simulink model "uniqueWordMethod"  (R2018b)
settings: Solver=FixedStepDiscrete  StartTime=0.0  StopTime=1000  RelTol=1e-3
libraries: simulink x2, commutil2 x2, commdigbbndpm3 x2, commfilt2 x2, dspstat3 x1, commrandsrc3 x1, commsink2 x1, commrflib2 x1, dspsigops x1
settings Model: Creator=sikor  LastModifiedBy=sikor
settings OptimizationCC: LifeSpan=inf
settings DebuggingCC: SFUnexpectedBacktrackingDiag=warning  SFNoUnconditionalDefaultTransitionDiag=warning
settings SFSimCC: SimUseLocalCustomCode=off
settings RTWCC: RTWUseLocalCustomCode=off
settings CodeAppCC: StateflowObjectComments=on
settings GRTTargetCC: TargetLangStandard=C89/C90 (ANSI)  GeneratePreprocessorConditionals=Disable all
settings ConfigComp: CovMetricSettings=dw  CovHtmlReporting=on  CovSaveCumulativeToWorkspaceVar=on  CovSaveSingleToWorkspaceVar=on  CovExternalEMLEnable=off

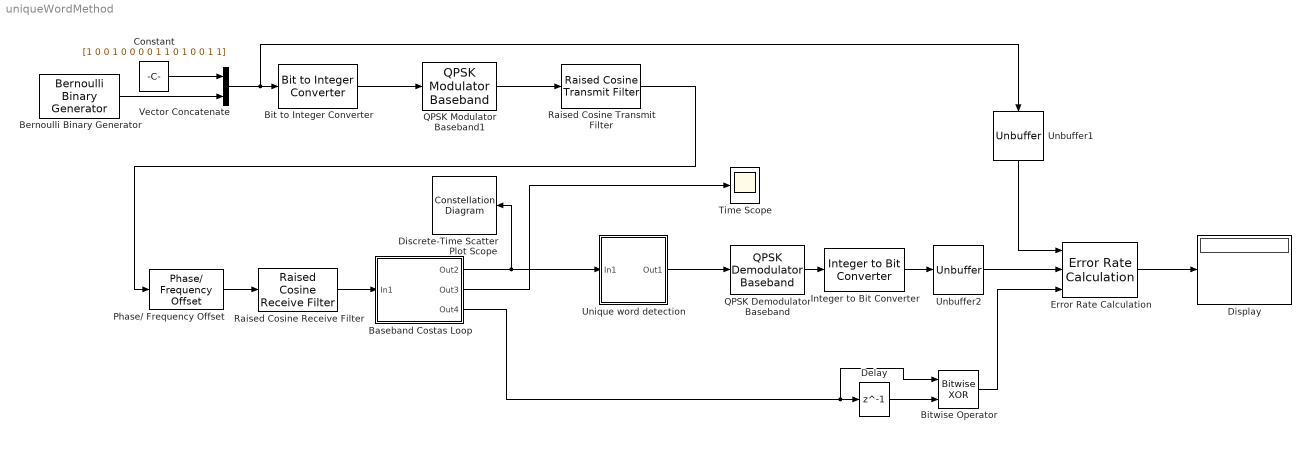
== system uniqueWordMethod ==
  Baseband Costas Loop : Subsystem  mask{loopBw=2.0*pi/100.0, sampleTime=1}
      mask prompts: loopBw "Select loop bandwidth"; sampleTime "Sample time"
      mask init:
      | damp=0.707;
      | %set_param('costasLoop','AlgebraicLoopSolver','TrustRegion')
      | alpha = (4.0 * damp * loopBw) / (1.0 + 2.0 * damp * loopBw + loopBw * loopBw); 
      | beta = (4.0 * loopBw * loopBw) / (1.0 + 2.0 * damp * loopBw + loopBw * loopBw); 
      | set_param(sprintf('%s/Baseband Costas Loop/Alfa',gcs),'Gain',sprintf('%f',alpha))
      | set_param(sprintf('%s/Baseband Costas Loop/Beta',gcs),'Gain',sprintf('%f',beta))
      | %set_param(sprintf('%s/Baseband Costas Loop/Mean1',gcs),'Ts',sprintf('%f',sampleTime))
      mask Display: disp('Costas\nLoop');
  Bernoulli Binary Generator : commrandsrc3/Bernoulli Binary Generator  ProbabilityOfZero=0.5  SeedSource=Auto  Seed=0  SampleTime=128  SamplesPerFrame=240  OutputDataType=uint8  SimulateUsing=Interpreted execution
      settings: SourceProductName=Communications Toolbox
  Bit to Integer Converter : commutil2/Bit to Integer Converter  nbits=2  bitOrder=MSB first  signedOutputValues=Unsigned  outDtype=int16  outDtypeSigned=Inherit via internal rule
      settings: SourceProductName=Communications Toolbox
  Bitwise Operator : simulink/Logic and Bit Operations/Bitwise Operator  logicop=XOR  UseBitMask=off  NumInputPorts=2  BitMask=bin2dec('11011001')  BitMaskRealWorld=Stored Integer
  Constant : Constant  Value=[1 0 0 1 0 0 0 0 1 1 0 1 0 0 1 1]  OutDataTypeStr=uint8  SampleTime=128
  Delay : Delay  DelayLength=1  InitialCondition=0
  Discrete-Time Scatter Plot Scope : ConstellationDiagram  Tag=ScatterPlot
  Display : Display
  Error Rate Calculation : commsink2/Error Rate Calculation  N=276  st_delay=0  cp_mode=Entire frame  subframe=[]  PMode=Port  WsName=ErrorVec  RsMode2=on  stop=off  numErr=100  maxBits=1e6
      settings: SourceProductName=Communications Toolbox
  Integer to Bit Converter : commutil2/Integer to Bit Converter  nbits=2  signedInputValues=Unsigned  bitOrder=MSB first  outDtype=Inherit via internal rule
      settings: SourceProductName=Communications Toolbox
  Phase/ Frequency Offset : commrflib2/Phase// Frequency Offset  phaseOffset=40  freqPort=off  freqOffset=.0000000000000000045
      settings: SourceProductName=Communications Toolbox
  QPSK Demodulator Baseband : commdigbbndpm3/QPSK Demodulator Baseband  OutType=Integer  DecType=Hard decision  VarSource=Dialog  Variance=1  Dec=Gray  Ph=pi/4  outDtype1=Inherit via internal rule  outDtype2=int16  derotateFactorWordLen=16  derotateFactorDataTypeStr=Inherit: Same word length as input  derotateFactorLastDataTypeStr=Inherit: Same word length as input
      settings: SourceProductName=Communications Toolbox
  QPSK Modulator Baseband1 : commdigbbndpm3/QPSK Modulator Baseband  InType=Integer  Enc=Gray  Ph=pi/4  outDtype=double  outWordLen=16  outUDDataType=sfix(16)  outFracLenMode=Best precision  outFracLen=15  outDataTypeStr=double  outLastDataTypeStr=double
      settings: SourceProductName=Communications Toolbox
  Raised Cosine Receive Filter : commfilt2/Raised Cosine Receive Filter  filtType=Square root  R=0.2  filtSpan=10  N=4  downFactor=4  downOffset=0  filterGain=1  InputProcessing=Columns as channels (frame based)  RateOptions=Allow multirate processing  framing=Mute  checkCoeff=off  variableName=rcRxFilt  currentFiltSpan=10  D=5  inputOffset=0  sampMode=Mute  saveAsFlag=0  rateMode=Downsampling  checkGain=Normalized  launchFVT=on  roundingMode=Floor  overflowMode=off  coeffDataTypeStr=Inherit: Same word length as input  coeffMin=[]  coeffMax=[]  coeffLastDataTypeStr=Inherit: Same word length as input  accumDataTypeStr=Inherit: Same as product output  accumLastDataTypeStr=Inherit: Same as product output  outputDataTypeStr=Inherit: Same as accumulator  outputMin=[]  outputMax=[]  outputLastDataTypeStr=Inherit: Same as accumulator
      settings: SourceProductName=Communications Toolbox
  Raised Cosine Transmit Filter : commfilt2/Raised Cosine Transmit Filter  filtType=Square root  R=0.2  filtSpan=10  N=4  filterGain=1  InputProcessing=Columns as channels (frame based)  RateOptions=Allow multirate processing  framing=Mute  checkCoeff=off  variableName=rcTxFilt  checkGain=Normalized  sampMode=Mute  saveAsFlag=0  currentFiltSpan=10  D=5  launchFVT=on  roundingMode=Floor  overflowMode=off  coeffDataTypeStr=Inherit: Same word length as input  coeffMin=[]  coeffMax=[]  coeffLastDataTypeStr=Inherit: Same word length as input  outputDataTypeStr=Inherit: Same as accumulator  outputMin=[]  outputMax=[]  outputLastDataTypeStr=Inherit: Same as accumulator
      settings: SourceProductName=Communications Toolbox
  Time Scope : Scope
  Unbuffer1 : Unbuffer
  Unbuffer2 : Unbuffer
  Unique word detection : Subsystem
      mask Display: disp('Detect phase\nshift')
  Vector Concatenate : Concatenate
  wires:
  Constant/1 -> Vector Concatenate/1
  Bernoulli Binary Generator/1 -> Vector Concatenate/2
  Vector Concatenate/1 -> Unbuffer1/1, Bit to Integer Converter/1
  Raised Cosine Transmit Filter/1 -> Phase/ Frequency Offset/1
  QPSK Modulator Baseband1/1 -> Raised Cosine Transmit Filter/1
  Bit to Integer Converter/1 -> QPSK Modulator Baseband1/1
  Error Rate Calculation/1 -> Display/1
  Phase/ Frequency Offset/1 -> Raised Cosine Receive Filter/1
  Raised Cosine Receive Filter/1 -> Baseband Costas Loop/1(In1)
  Baseband Costas Loop/2(Out3) -> Time Scope/1
  Delay/1 -> Bitwise Operator/2
  Baseband Costas Loop/3(Out4) -> Delay/1, Bitwise Operator/1
  Bitwise Operator/1 -> Error Rate Calculation/3
  Baseband Costas Loop/1(Out2) -> Unique word detection/1(In1), Discrete-Time Scatter Plot Scope/1
  Unique word detection/1(Out1) -> QPSK Demodulator Baseband/1
  QPSK Demodulator Baseband/1 -> Integer to Bit Converter/1
  Unbuffer1/1 -> Error Rate Calculation/1
  Integer to Bit Converter/1 -> Unbuffer2/1
  Unbuffer2/1 -> Error Rate Calculation/2

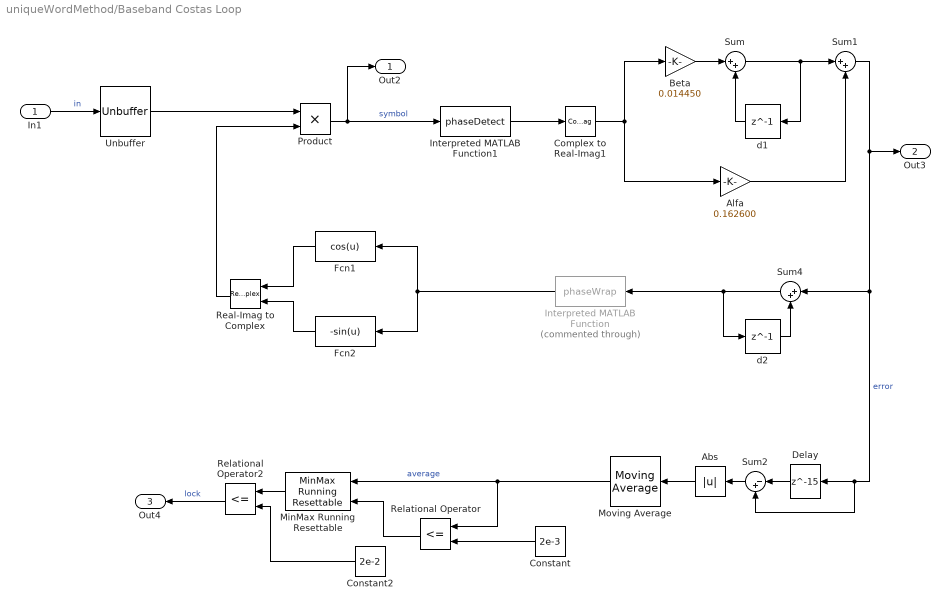
== system uniqueWordMethod/Baseband Costas Loop ==
  In1 : Inport
  Abs : Abs
  Alfa : Gain  Gain=0.162600
  Beta : Gain  Gain=0.014450
  Complex to Real-Imag1 : ComplexToRealImag  Output=Real
  Constant : Constant  Value=2e-3
  Constant2 : Constant  Value=2e-2
  Delay : Delay  DelayLength=15  InitialCondition=0
  Fcn1 : Fcn  Expr=cos(u)
  Fcn2 : Fcn  Expr=-sin(u)
  Interpreted MATLAB Function : MATLABFcn  Commented=through  MATLABFcn=phaseWrap
  Interpreted MATLAB Function1 : MATLABFcn  MATLABFcn=phaseDetect
  MinMax Running Resettable : simulink/Math Operations/MinMax Running Resettable  Function=max  vinit=0.0
  Moving Average : dspstat3/Moving Average  Method=Sliding window  ForgettingFactorPort=off  SpecifyWindowLength=on  WindowLength=64  ForgettingFactor=0.9  SimulateUsing=Code generation
  Product : Product  OutDataTypeStr=double  RndMeth=Round
  Real-Imag to Complex : RealImagToComplex
  Relational Operator : RelationalOperator  Operator=<=  OutDataTypeStr=boolean  RndMeth=Nearest
  Relational Operator2 : RelationalOperator  Operator=<=  OutDataTypeStr=boolean  RndMeth=Nearest
  Sum : Sum  Inputs=|++  OutDataTypeStr=double  RndMeth=Round
  Sum1 : Sum  Inputs=|++  OutDataTypeStr=double  RndMeth=Nearest
  Sum2 : Sum  Inputs=|-+
  Sum4 : Sum  Inputs=|++
  Unbuffer : Unbuffer
  d1 : Delay  DelayLength=1  InitialCondition=0
  d2 : Delay  DelayLength=1  InitialCondition=0
  Out2 : Outport
  Out3 : Outport  Port=2
  Out4 : Outport  Port=3
  wires:
  In1/1 -> Unbuffer/1  "in"
  d1/1 -> Sum/2
  Sum/1 -> d1/1, Sum1/1
  Alfa/1 -> Sum1/2
  Beta/1 -> Sum/1
  Product/1 -> Out2/1, Interpreted MATLAB Function1/1  "symbol"
  Real-Imag to Complex/1 -> Product/2
  Unbuffer/1 -> Product/1
  Sum4/1 -> d2/1, Interpreted MATLAB Function/1
  d2/1 -> Sum4/2
  Interpreted MATLAB Function/1 -> Fcn1/1, Fcn2/1
  Fcn1/1 -> Real-Imag to Complex/1
  Fcn2/1 -> Real-Imag to Complex/2
  Sum1/1 -> Sum2/2, Delay/1, Sum4/1, Out3/1  "error"
  Interpreted MATLAB Function1/1 -> Complex to Real-Imag1/1
  Complex to Real-Imag1/1 -> Alfa/1, Beta/1
  Constant2/1 -> Relational Operator2/2
  Delay/1 -> Sum2/1
  Constant/1 -> Relational Operator/2
  Sum2/1 -> Abs/1
  Moving Average/1 -> MinMax Running Resettable/1, Relational Operator/1  "average"
  Relational Operator/1 -> MinMax Running Resettable/2
  MinMax Running Resettable/1 -> Relational Operator2/1
  Abs/1 -> Moving Average/1
  Relational Operator2/1 -> Out4/1  "lock"

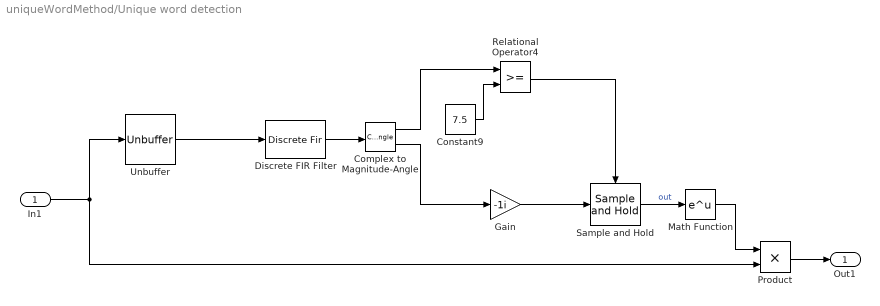
== system uniqueWordMethod/Unique word detection ==
  In1 : Inport
  Complex to Magnitude-Angle : ComplexToMagnitudeAngle
  Constant9 : Constant  Value=7.5
  Discrete FIR Filter : DiscreteFir  Coefficients=[-0.7071 + 0.7071i; 0.7071 - 0.7071i; -0.7071 - 0.7071i ;-0.7071 + 0.7071i; 0.7071 - 0.7071i; 0.7071 - 0.7071i ;-0.7071 - 0.7071i; 0.7071 + 0.7071i].'
  Gain : Gain  Gain=-1i
  Math Function : Math  SaturateOnIntegerOverflow=on
  Product : Product
  Relational Operator4 : RelationalOperator  OutDataTypeStr=boolean  RndMeth=Nearest
  Sample and Hold : dspsigops/Sample and Hold  trig=Rising edge  initCond=0  latchinput=off
  Unbuffer : Unbuffer
  Out1 : Outport
  wires:
  Relational Operator4/1 -> Sample and Hold/Trigger
  Constant9/1 -> Relational Operator4/2
  In1/1 -> Unbuffer/1, Product/2
  Discrete FIR Filter/1 -> Complex to Magnitude-Angle/1
  Complex to Magnitude-Angle/1 -> Relational Operator4/1
  Complex to Magnitude-Angle/2 -> Gain/1
  Gain/1 -> Sample and Hold/1
  Sample and Hold/1 -> Math Function/1  "out"
  Math Function/1 -> Product/1
  Product/1 -> Out1/1
  Unbuffer/1 -> Discrete FIR Filter/1
